simulink model "RateAdaptiveWereBack"  (R2023b)
settings: Solver=FixedStepAuto  StartTime=0.0  StopTime=300  FixedStep=1e-3  RelTol=1e-3  EnableMultiTasking=on
undefined symbols (not defined in the file or in its folder): D0, D1, D10, D11, D12, D13, D2, D3, D4, D5, D6, D7, D8, D9, PTA0, PTA1, PTA2, PTB23, PTB9, PTC16, PTC17, PTC2, PTC3, PTC4, PTD0, PTD1, PTD2, PTD3
libraries: frdmk64flib x15, dspstat3 x1
settings Model: SimulationMode=external  PacingRate=0.250000  ExtModeTrigDuration=5  Creator=mathewgaluszka  LastModifiedBy=Mathew
settings OptimizationCC: EnhancedBackFolding=on  PassReuseOutputArgsAs=Individual arguments  ZeroExternalMemoryAtStartup=off  ZeroInternalMemoryAtStartup=off  MaxStackSize=64  OptimizeBlockOrder=speed  DifferentSizesBufferReuse=on  OptimizationCustomize=off  EfficientTunableParamExpr=on
settings DebuggingCC: ParameterTunabilityLossMsg=error
settings HardwareCC: ProdBitPerPointer=32  ProdBitPerSizeT=32  ProdBitPerPtrDiffT=32  ProdLargestAtomicInteger=Long  ProdLargestAtomicFloat=Double  ProdWordSize=32  ProdHWDeviceType=ARM Compatible->ARM Cortex
settings SFSimCC: MATLABDynamicMemAlloc=off
settings RTWCC: Description=Embedded Coder  SystemTargetFile=ert.tlc  HardwareBoard=NXP FRDM-K64F  TLCOptions="-aInlineSetEventsForThisBaseRateFcn=TLC_FALSE -aSuppressMultiTaskScheduler=TLC_FALSE  -aRateBasedStepFcn=0"  TemplateMakefile=ert_default_tmf  Toolchain=GNU Tools for ARM Embedded Processors
settings CodeAppCC: ForceParamTrailComments=on  IgnoreCustomStorageClasses=off  OperatorAnnotations=on  SimulinkDataObjDesc=on  SFDataObjDesc=on  InsertBlockDesc=on
settings ERTTargetCC: SupportContinuousTime=on  ExtMode=on  ExtModeTransport=4  ExtModeMexFile=sendToCommService  ExtModeMexArgs='RateAdaptive' 0

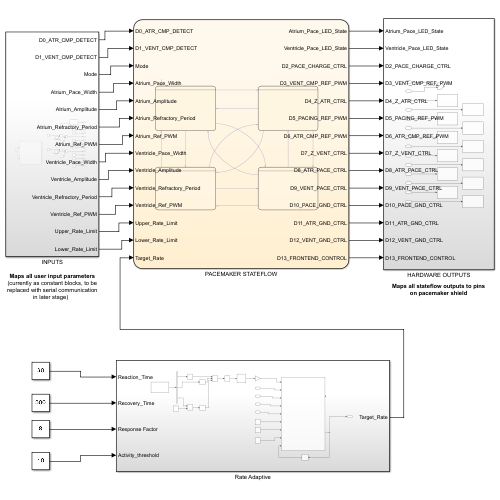
[thumbnail: Simulink's stored preview of the top-level diagram]
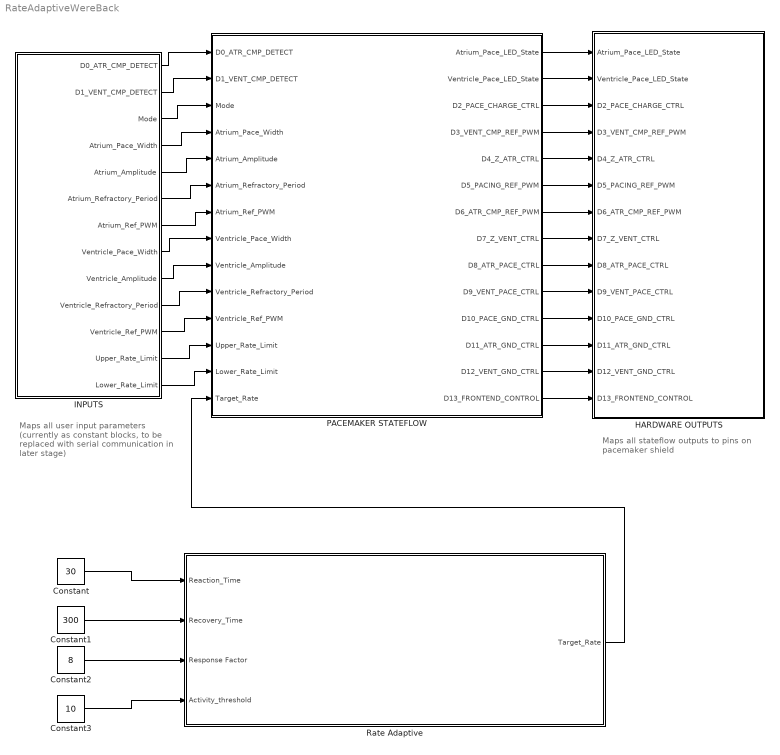
== system RateAdaptiveWereBack ==
  note: Maps all user input parameters (currently as constant blocks, to be replaced with serial communication in later stage)
  note: Maps all stateflow outputs to pins on pacemaker shield
  Constant : Constant  Value=30
  Constant1 : Constant  Value=300
  Constant2 : Constant  Value=8
  Constant3 : Constant  Value=10
  HARDWARE OUTPUTS : Subsystem
  INPUTS : Subsystem
  PACEMAKER STATEFLOW : Stateflow chart  TreatAsAtomicUnit=on
  Rate Adaptive : Subsystem
  wires:
  PACEMAKER STATEFLOW/1(Atrium_Pace_LED_State) -> HARDWARE OUTPUTS/1(Atrium_Pace_LED_State)
  PACEMAKER STATEFLOW/2(Ventricle_Pace_LED_State) -> HARDWARE OUTPUTS/2(Ventricle_Pace_LED_State)
  PACEMAKER STATEFLOW/3(D2_PACE_CHARGE_CTRL) -> HARDWARE OUTPUTS/3(D2_PACE_CHARGE_CTRL)
  PACEMAKER STATEFLOW/4(D3_VENT_CMP_REF_PWM) -> HARDWARE OUTPUTS/4(D3_VENT_CMP_REF_PWM)
  PACEMAKER STATEFLOW/5(D4_Z_ATR_CTRL) -> HARDWARE OUTPUTS/5(D4_Z_ATR_CTRL)
  PACEMAKER STATEFLOW/6(D5_PACING_REF_PWM) -> HARDWARE OUTPUTS/6(D5_PACING_REF_PWM)
  PACEMAKER STATEFLOW/7(D6_ATR_CMP_REF_PWM) -> HARDWARE OUTPUTS/7(D6_ATR_CMP_REF_PWM)
  PACEMAKER STATEFLOW/8(D7_Z_VENT_CTRL) -> HARDWARE OUTPUTS/8(D7_Z_VENT_CTRL)
  PACEMAKER STATEFLOW/9(D8_ATR_PACE_CTRL) -> HARDWARE OUTPUTS/9(D8_ATR_PACE_CTRL)
  PACEMAKER STATEFLOW/10(D9_VENT_PACE_CTRL) -> HARDWARE OUTPUTS/10(D9_VENT_PACE_CTRL)
  PACEMAKER STATEFLOW/11(D10_PACE_GND_CTRL) -> HARDWARE OUTPUTS/11(D10_PACE_GND_CTRL)
  PACEMAKER STATEFLOW/12(D11_ATR_GND_CTRL) -> HARDWARE OUTPUTS/12(D11_ATR_GND_CTRL)
  PACEMAKER STATEFLOW/13(D12_VENT_GND_CTRL) -> HARDWARE OUTPUTS/13(D12_VENT_GND_CTRL)
  PACEMAKER STATEFLOW/14(D13_FRONTEND_CONTROL) -> HARDWARE OUTPUTS/14(D13_FRONTEND_CONTROL)
  INPUTS/1(D0_ATR_CMP_DETECT) -> PACEMAKER STATEFLOW/1(D0_ATR_CMP_DETECT)
  INPUTS/2(D1_VENT_CMP_DETECT) -> PACEMAKER STATEFLOW/2(D1_VENT_CMP_DETECT)
  INPUTS/3(Mode) -> PACEMAKER STATEFLOW/3(Mode)
  INPUTS/4(Atrium_Pace_Width) -> PACEMAKER STATEFLOW/4(Atrium_Pace_Width)
  INPUTS/5(Atrium_Amplitude) -> PACEMAKER STATEFLOW/5(Atrium_Amplitude)
  INPUTS/6(Atrium_Refractory_Period) -> PACEMAKER STATEFLOW/6(Atrium_Refractory_Period)
  INPUTS/7(Atrium_Ref_PWM) -> PACEMAKER STATEFLOW/7(Atrium_Ref_PWM)
  INPUTS/8(Ventricle_Pace_Width) -> PACEMAKER STATEFLOW/8(Ventricle_Pace_Width)
  INPUTS/9(Ventricle_Amplitude) -> PACEMAKER STATEFLOW/9(Ventricle_Amplitude)
  INPUTS/10(Ventricle_Refractory_Period) -> PACEMAKER STATEFLOW/10(Ventricle_Refractory_Period)
  INPUTS/11(Ventricle_Ref_PWM) -> PACEMAKER STATEFLOW/11(Ventricle_Ref_PWM)
  INPUTS/12(Upper_Rate_Limit) -> PACEMAKER STATEFLOW/12(Upper_Rate_Limit)
  INPUTS/13(Lower_Rate_Limit) -> PACEMAKER STATEFLOW/13(Lower_Rate_Limit)
  Constant/1 -> Rate Adaptive/1(Reaction_Time)
  Constant2/1 -> Rate Adaptive/3(Response Factor)
  Constant3/1 -> Rate Adaptive/4(Activity_threshold)
  Constant1/1 -> Rate Adaptive/2(Recovery_Time)
  Rate Adaptive/1(Target_Rate) -> PACEMAKER STATEFLOW/14(Target_Rate)

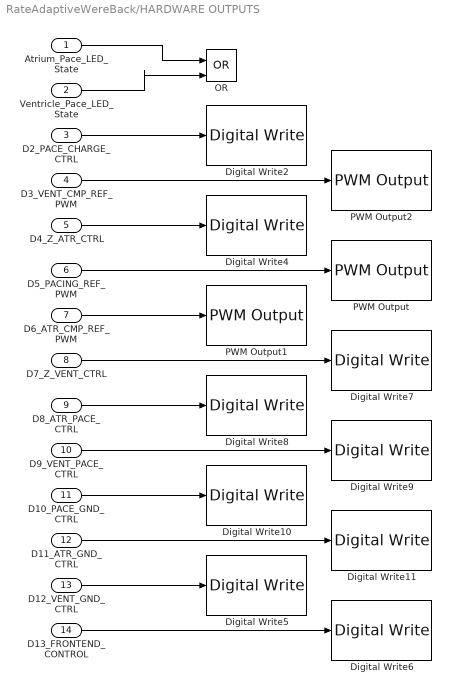
== system RateAdaptiveWereBack/HARDWARE OUTPUTS ==
  Atrium_Pace_LED_State : Inport
  Ventricle_Pace_LED_State : Inport  Port=2
  D2_PACE_CHARGE_CTRL : Inport  Port=3
  D3_VENT_CMP_REF_PWM : Inport  Port=4
  D4_Z_ATR_CTRL : Inport  Port=5
  D5_PACING_REF_PWM : Inport  Port=6
  D6_ATR_CMP_REF_PWM : Inport  Port=7
  D7_Z_VENT_CTRL : Inport  Port=8
  D8_ATR_PACE_CTRL : Inport  Port=9
  D9_VENT_PACE_CTRL : Inport  Port=10
  D10_PACE_GND_CTRL : Inport  Port=11
  D11_ATR_GND_CTRL : Inport  Port=12
  D12_VENT_GND_CTRL : Inport  Port=13
  D13_FRONTEND_CONTROL : Inport  Port=14
  Digital Write10 : frdmk64flib/Digital Write  Whichpin=PTD0 (D10)
  Digital Write11 : frdmk64flib/Digital Write  Whichpin=PTD2 (D11)
  Digital Write2 : frdmk64flib/Digital Write  Whichpin=PTB9 (D2)
  Digital Write4 : frdmk64flib/Digital Write  Whichpin=PTB23 (D4)
  Digital Write5 : frdmk64flib/Digital Write  Whichpin=PTD3 (D12)
  Digital Write6 : frdmk64flib/Digital Write  Whichpin=PTD1 (D13)
  Digital Write7 : frdmk64flib/Digital Write  Whichpin=PTC3 (D7)
  Digital Write8 : frdmk64flib/Digital Write  Whichpin=PTA0 (D8)
  Digital Write9 : frdmk64flib/Digital Write  Whichpin=PTC4 (D9)
  OR : Logic  Operator=OR  IconShape=distinctive  AllPortsSameDT=off  OutDataTypeStr=boolean
  PWM Output : frdmk64flib/PWM Output  Whichpin=PTA2 (D5)  InitialFrequency=2000  InitialDutyCycle=0
  PWM Output1 : frdmk64flib/PWM Output  Whichpin=PTC2 (D6)  InitialFrequency=2000  InitialDutyCycle=0
  PWM Output2 : frdmk64flib/PWM Output  Whichpin=PTA1 (D3)  InitialFrequency=2000  InitialDutyCycle=0
  wires:
  D2_PACE_CHARGE_CTRL/1 -> Digital Write2/1
  D3_VENT_CMP_REF_PWM/1 -> PWM Output2/1
  D4_Z_ATR_CTRL/1 -> Digital Write4/1
  D5_PACING_REF_PWM/1 -> PWM Output/1
  D6_ATR_CMP_REF_PWM/1 -> PWM Output1/1
  D7_Z_VENT_CTRL/1 -> Digital Write7/1
  D8_ATR_PACE_CTRL/1 -> Digital Write8/1
  D9_VENT_PACE_CTRL/1 -> Digital Write9/1
  D10_PACE_GND_CTRL/1 -> Digital Write10/1
  D11_ATR_GND_CTRL/1 -> Digital Write11/1
  D12_VENT_GND_CTRL/1 -> Digital Write5/1
  D13_FRONTEND_CONTROL/1 -> Digital Write6/1
  Atrium_Pace_LED_State/1 -> OR/1
  Ventricle_Pace_LED_State/1 -> OR/2

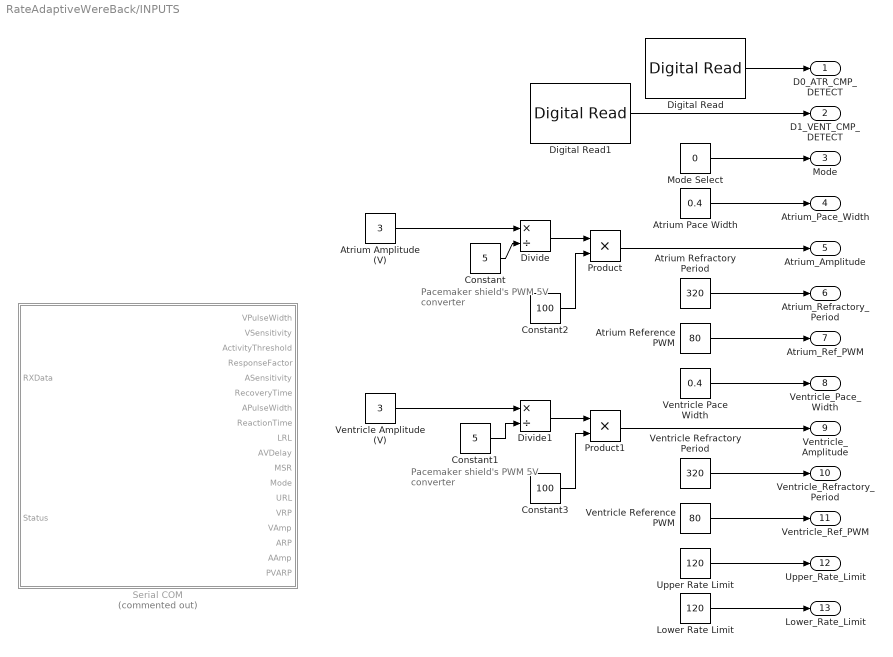
== system RateAdaptiveWereBack/INPUTS ==
  note: Pacemaker shield's PWM 5V converter
  note: Pacemaker shield's PWM 5V converter
  Atrium Amplitude (V) : Constant  Value=3
  Atrium Pace Width : Constant  Value=0.4
  Atrium Reference PWM : Constant  Value=80
  Atrium Refractory Period : Constant  Value=320
  Constant : Constant  Value=5
  Constant1 : Constant  Value=5
  Constant2 : Constant  Value=100
  Constant3 : Constant  Value=100
  Digital Read : frdmk64flib/Digital Read  Whichpin=PTC16 (D0)  SampleTime=-1
  Digital Read1 : frdmk64flib/Digital Read  Whichpin=PTC17 (D1)  SampleTime=-1
  Divide : Product  Inputs=*/
  Divide1 : Product  Inputs=*/
  Lower Rate Limit : Constant  Value=120
  Mode Select : Constant  Value=0
  Product : Product
  Product1 : Product
  Serial COM : Stateflow chart  Commented=on  TreatAsAtomicUnit=on
  Upper Rate Limit : Constant  Value=120
  Ventricle Amplitude (V) : Constant  Value=3
  Ventricle Pace Width : Constant  Value=0.4
  Ventricle Reference PWM : Constant  Value=80
  Ventricle Refractory Period : Constant  Value=320
  D0_ATR_CMP_DETECT : Outport
  D1_VENT_CMP_DETECT : Outport  Port=2
  Mode : Outport  Port=3
  Atrium_Pace_Width : Outport  Port=4
  Atrium_Amplitude : Outport  Port=5
  Atrium_Refractory_Period : Outport  Port=6
  Atrium_Ref_PWM : Outport  Port=7
  Ventricle_Pace_Width : Outport  Port=8
  Ventricle_Amplitude : Outport  Port=9
  Ventricle_Refractory_Period : Outport  Port=10
  Ventricle_Ref_PWM : Outport  Port=11
  Upper_Rate_Limit : Outport  Port=12
  Lower_Rate_Limit : Outport  Port=13
  wires:
  Digital Read/1 -> D0_ATR_CMP_DETECT/1
  Digital Read1/1 -> D1_VENT_CMP_DETECT/1
  Mode Select/1 -> Mode/1
  Atrium Pace Width/1 -> Atrium_Pace_Width/1
  Atrium Refractory Period/1 -> Atrium_Refractory_Period/1
  Atrium Reference PWM/1 -> Atrium_Ref_PWM/1
  Ventricle Pace Width/1 -> Ventricle_Pace_Width/1
  Ventricle Refractory Period/1 -> Ventricle_Refractory_Period/1
  Ventricle Reference PWM/1 -> Ventricle_Ref_PWM/1
  Upper Rate Limit/1 -> Upper_Rate_Limit/1
  Lower Rate Limit/1 -> Lower_Rate_Limit/1
  Atrium Amplitude (V)/1 -> Divide/1
  Constant/1 -> Divide/2
  Ventricle Amplitude (V)/1 -> Divide1/1
  Constant1/1 -> Divide1/2
  Divide/1 -> Product/1
  Product/1 -> Atrium_Amplitude/1
  Constant2/1 -> Product/2
  Divide1/1 -> Product1/1
  Product1/1 -> Ventricle_Amplitude/1
  Constant3/1 -> Product1/2
  ? -> Serial COM/1(RXData)
  ? -> Serial COM/2(Status)

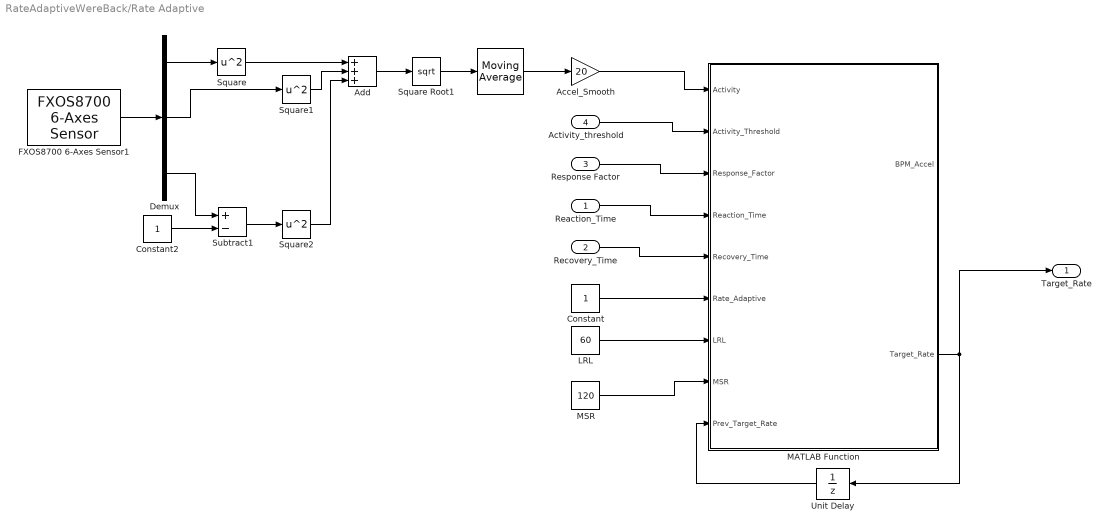
== system RateAdaptiveWereBack/Rate Adaptive ==
  Reaction_Time : Inport
  Recovery_Time : Inport  Port=2
  Response Factor : Inport  Port=3
  Activity_threshold : Inport  Port=4
  " " : dspstat3/Moving Average  Method=Sliding window  ForgettingFactorPort=off  SpecifyWindowLength=on  WindowLength=300  OverlapLength=299  AllowArbitraryInputLength=off  ForgettingFactor=0.9  SimulateUsing=Code generation
  Accel_Smooth : Gain  Gain=20
  Add : Sum  Inputs=+++
  Constant : Constant
  Constant2 : Constant
  Demux : Demux  Outputs=3
  FXOS8700 6-Axes Sensor1 : frdmk64flib/FXOS8700 6-Axes Sensor  Activesensor=Accelerometer only  ODR=800Hz  HybridODR=400Hz  Accelfullrange=-4g to +4g  SampleTime=-1
  LRL : Constant  Value=60
  MATLAB Function : MATLAB Function  TreatAsAtomicUnit=on
  MSR : Constant  Value=120
  Square : Math  Operator=square
  Square Root1 : Sqrt
  Square1 : Math  Operator=square
  Square2 : Math  Operator=square
  Subtract1 : Sum  Inputs=+-
  Unit Delay : UnitDelay  SampleTime=-1  HasFrameUpgradeWarning=on
  Target_Rate : Outport
  wires:
  Constant/1 -> MATLAB Function/6(Rate_Adaptive)
  FXOS8700 6-Axes Sensor1/1 -> Demux/1
  Demux/1 -> Square/1
  Square1/1 -> Add/2
  Square/1 -> Add/1
  Demux/2 -> Square1/1
  Demux/3 -> Subtract1/1
  Constant2/1 -> Subtract1/2
  Subtract1/1 -> Square2/1
  Square2/1 -> Add/3
  Add/1 -> Square Root1/1
  Square Root1/1 -> " "/1
  " "/1 -> Accel_Smooth/1
  Accel_Smooth/1 -> MATLAB Function/1(Activity)
  Activity_threshold/1 -> MATLAB Function/2(Activity_Threshold)
  Recovery_Time/1 -> MATLAB Function/5(Recovery_Time)
  Response Factor/1 -> MATLAB Function/3(Response_Factor)
  LRL/1 -> MATLAB Function/7(LRL)
  Reaction_Time/1 -> MATLAB Function/4(Reaction_Time)
  MSR/1 -> MATLAB Function/8(MSR)
  MATLAB Function/2(Target_Rate) -> Unit Delay/1, Target_Rate/1
  Unit Delay/1 -> MATLAB Function/9(Prev_Target_Rate)

== stateflow chart RateAdaptiveWereBack/INPUTS/Serial COM ==
  state Preset
    entry:
    Mode=0;   %int unit8
    LRL=60;   %BPM uint8
    URL=120;   %BPM uint8
    MSR=120;   %BPM uint8
    AVDelay=150;   %ms uint8
    AAmp=3.5;   %V single
    VAmp=3.5;   %V single
    APulseWidth=0.4;   %ms single
    VPulseWidth=0.4;   %ms single
    ASensitivity=0.75;   %mV single
    VSensitivity=2.5;   %mV single
    ARP=250;   %ms uint16
    VRP=320;   %ms uint16
    PVARP=250;   %ms uint16
    ActivityThreshold=4;   %int uint8
    ReactionTime=30;   %s uint8
    ResponseFactor=8   %int uint8
    RecoveryTime=5;   %min uint8
  state SaveData
    entry:
    Mode=RXData(3);   %int unit8
    LRL=RXData(4);   %BPM uint8
    URL=RXData(5);   %BPM uint8
    MSR=RXData(6);   %BPM uint8
    AVDelay=RXData(7);   %ms uint8
    AAmp=RXData(8:11);   %V single
    VAmp=RXData(12:15);   %V single
    APulseWidth=RXData(16:19);   %ms single
    VPulseWidth=RXData(20:23);   %ms single
    ASensitivity=RXData(24:27);   %mV single
    VSensitivity=RXData(28:31);   %mV single
    ARP=RXData(32:33);   %ms uint16
    VRP=RXData(34:35);   %ms uint16
    PVARP=RXData(36:37);   %ms uint16
    ActivityThreshold=RXData(38);   %int uint8
    ReactionTime=RXData(39);   %s uint8
    ResponseFactor=RXData(40)   %int uint8
    RecoveryTime=RXData(41);   %min uint8
  state Standby
  state CheckSync
  state CheckFunction
  state ReturnData
  (default) -> Preset
  CheckSync -> Standby [order 2]
  Standby -> CheckSync : [Status==0]
  Preset -> Standby
  CheckFunction -> SaveData [order 2] : [RXData(2)==hex2dec('22')]
  CheckSync -> CheckFunction [order 1] : [RXData(1)==hex2dec('16')]
  ReturnData -> Standby
  SaveData -> Standby
  CheckFunction -> ReturnData [order 1] : [RXData(2)==hex2dec('22')]
  data: RXData input; Status input; VPulseWidth output; VSensitivity output; ActivityThreshold output; ResponseFactor output; ASensitivity output; RecoveryTime output; APulseWidth output; ReactionTime output; LRL output; AVDelay output; MSR output; Mode output; URL output; VRP output; VAmp output; ARP output; AAmp output; PVARP output

== matlab function RateAdaptiveWereBack/Rate Adaptive/MATLAB Function ==
  data: Activity input; Activity_Threshold input; BPM_Accel output; Response_Factor input; Reaction_Time input; Recovery_Time input; Rate_Adaptive input; LRL input; MSR input; Prev_Target_Rate input; Target_Rate output
function [BPM_Accel,Target_Rate]  = Rate_Response(Activity,Activity_Threshold,Response_Factor,Reaction_Time,Recovery_Time,Rate_Adaptive,LRL,MSR,Prev_Target_Rate)

Activity_Factor = 10*Response_Factor*(Activity-Activity_Threshold);

derivative_Activity=diff(Activity);

if(Rate_Adaptive==0)
    BPM_Accel=0;
elseif(derivative_Activity>=0)
    BPM_Accel=Activity_Factor/Reaction_Time;
else
    BPM_Accel=Activity_Factor/Recovery_Time;
end

Target_Rate=BPM_Accel*(1e-3)+Prev_Target_Rate;

if(Target_Rate<LRL)
    Target_Rate=LRL;
elseif(Target_Rate>MSR)
    Target_Rate=MSR;
end

== stateflow chart RateAdaptiveWereBack/PACEMAKER STATEFLOW ==
  state AOO
    state Pace
      entry:
      D5_PACING_REF_PWM = 0
      D2_PACE_CHARGE_CTRL=0;
      D10_PACE_GND_CTRL=1;
      D8_ATR_PACE_CTRL=1;
      D11_ATR_GND_CTRL=0;
      D4_Z_ATR_CTRL=0;
      D7_Z_VENT_CTRL=0;
      D12_VENT_GND_CTRL=0;
      D9_VENT_PACE_CTRL=0;
      Atrium_Pace_LED_State=1;
    state Refractory
      entry:
      D10_PACE_GND_CTRL=1;
      D9_VENT_PACE_CTRL=0;
      D4_Z_ATR_CTRL=0;
      D7_Z_VENT_CTRL=0;
      D8_ATR_PACE_CTRL=0;
      D11_ATR_GND_CTRL=1;
      D12_VENT_GND_CTRL=0;
      D2_PACE_CHARGE_CTRL=1;
      D5_PACING_REF_PWM = Atrium_Amplitude
      Atrium_Pace_LED_State=0;
      Standby_Period=(1/(Target_Rate))*60000
    (default) -> AOO.Refractory
    AOO.Pace -> AOO.Refractory : [after(Atrium_Pace_Width,msec)]
    AOO.Refractory -> AOO.Pace : [after(Standby_Period,msec)]
  state AAI
    state Pace
      entry:
      D5_PACING_REF_PWM = 0
      D2_PACE_CHARGE_CTRL=0;
      D10_PACE_GND_CTRL=1;
      D8_ATR_PACE_CTRL=1;
      D11_ATR_GND_CTRL=0;
      D4_Z_ATR_CTRL=0;
      D7_Z_VENT_CTRL=0;
      D12_VENT_GND_CTRL=0;
      D9_VENT_PACE_CTRL=0;
      Atrium_Pace_LED_State=1;
    state Refractory
      entry:
      D5_PACING_REF_PWM = Atrium_Amplitude
      D10_PACE_GND_CTRL=1;
      D9_VENT_PACE_CTRL=0;
      D4_Z_ATR_CTRL=0;
      D7_Z_VENT_CTRL=0;
      D8_ATR_PACE_CTRL=0;
      D11_ATR_GND_CTRL=1;
      D12_VENT_GND_CTRL=0;
      D2_PACE_CHARGE_CTRL=1;
      D6_ATR_CMP_REF_PWM = Atrium_Ref_PWM;
      Atrium_Pace_LED_State=0;
      Standby_Period=60000/(Lower_Rate_Limit)
    state waiting
    state Sense
    AAI.Pace -> AAI.Refractory : [after(Atrium_Pace_Width,msec)]
    (default) -> AAI.Refractory
    AAI.waiting -> AAI.Sense : [[after(Atrium_Refractory_Period,msec)]]
    AAI.Refractory -> AAI.waiting
    AAI.Sense -> AAI.waiting [order 2] : [D0_ATR_CMP_DETECT == 1]
    AAI.Sense -> AAI.Pace [order 1] : after(Standby_Period-Atrium_Pace_Width-Atrium_Refractory_Period,msec)
  state VOO
    state Pace
      entry:
      D5_PACING_REF_PWM = 0
      D2_PACE_CHARGE_CTRL=0;
      D10_PACE_GND_CTRL=1;
      D8_ATR_PACE_CTRL=0;
      D11_ATR_GND_CTRL=0;
      D4_Z_ATR_CTRL=0;
      D7_Z_VENT_CTRL=0;
      D12_VENT_GND_CTRL=0;
      D9_VENT_PACE_CTRL=1;
      Ventricle_Pace_LED_State=1;
    state Refractory
      entry:
      D10_PACE_GND_CTRL=1;
      D9_VENT_PACE_CTRL=0;
      D4_Z_ATR_CTRL=0;
      D7_Z_VENT_CTRL=0;
      D8_ATR_PACE_CTRL=0;
      D11_ATR_GND_CTRL=0;
      D12_VENT_GND_CTRL=1;
      D2_PACE_CHARGE_CTRL=1;
      D5_PACING_REF_PWM = Ventricle_Amplitude
      Ventricle_Pace_LED_State=0;
      Standby_Period=(1/(Lower_Rate_Limit))*60000
    (default) -> VOO.Refractory
    VOO.Pace -> VOO.Refractory : [after(Ventricle_Pace_Width,msec)]
    VOO.Refractory -> VOO.Pace : [after(Standby_Period,msec)]
  state VVI
    state Pace
      entry:
      D5_PACING_REF_PWM = 0
      D2_PACE_CHARGE_CTRL=0;
      D10_PACE_GND_CTRL=1;
      D8_ATR_PACE_CTRL=0;
      D11_ATR_GND_CTRL=0;
      D4_Z_ATR_CTRL=0;
      D7_Z_VENT_CTRL=0;
      D12_VENT_GND_CTRL=0;
      D9_VENT_PACE_CTRL=1;
    state Refractory
      entry:
      D5_PACING_REF_PWM = Ventricle_Amplitude
      D10_PACE_GND_CTRL=1;
      D9_VENT_PACE_CTRL=0;
      D4_Z_ATR_CTRL=0;
      D7_Z_VENT_CTRL=0;
      D8_ATR_PACE_CTRL=0;
      D11_ATR_GND_CTRL=0;
      D12_VENT_GND_CTRL=1;
      D2_PACE_CHARGE_CTRL=1;
      D3_VENT_CMP_REF_PWM = Ventricle_Ref_PWM;
      Ventricle_Pace_LED_State=0;
      Standby_Period=60000/(Lower_Rate_Limit)
    state Sense
    state waiting
    VVI.Pace -> VVI.Refractory : [after(Ventricle_Pace_Width,msec)]
    (default) -> VVI.Refractory
    VVI.waiting -> VVI.Sense : [[after(Ventricle_Refractory_Period,msec)]]
    VVI.Refractory -> VVI.waiting
    VVI.Sense -> VVI.Pace [order 1] : after(Standby_Period-Ventricle_Pace_Width-Ventricle_Refractory_Period,msec)
    VVI.Sense -> VVI.waiting [order 2] : [D1_VENT_CMP_DETECT == 1]
  (default) -> AOO
  AOO -> AAI [order 1] : [Mode==2]
  AAI -> AOO [order 2] : [Mode==0]
  AOO -> VVI [order 3] : [Mode==3]
  VOO -> AAI [order 3] : [Mode==2]
  VOO -> AOO [order 1] : [Mode==0]
  AOO -> VOO [order 2] : [Mode==1]
  VVI -> AOO [order 3] : [Mode==0]
  AAI -> VOO [order 3] : [Mode==1]
  VVI -> AAI [order 2] : [Mode==2]
  AAI -> VVI [order 1] : [Mode==3]
  VOO -> VVI [order 2] : [Mode==3]
  VVI -> VOO [order 1] : [Mode==1]
  data: D0_ATR_CMP_DETECT input; D1_VENT_CMP_DETECT input; Mode input; Atrium_Pace_Width input; Atrium_Amplitude input; Atrium_Refractory_Period input; Atrium_Ref_PWM input; Ventricle_Pace_Width input; Ventricle_Amplitude input; Ventricle_Refractory_Period input; Ventricle_Ref_PWM input; Atrium_Pace_LED_State output; Ventricle_Pace_LED_State output; D2_PACE_CHARGE_CTRL output; D3_VENT_CMP_REF_PWM output; D4_Z_ATR_CTRL output; D5_PACING_REF_PWM output; D6_ATR_CMP_REF_PWM output; D7_Z_VENT_CTRL output; D8_ATR_PACE_CTRL output; D9_VENT_PACE_CTRL output; D10_PACE_GND_CTRL output; D11_ATR_GND_CTRL output; D12_VENT_GND_CTRL output; Upper_Rate_Limit input; Lower_Rate_Limit input; Standby_Period local; D13_FRONTEND_CONTROL output boolean =true; Target_Rate input
